simulink model "Disturbance"  (R2024b)
settings: Solver=FixedStepAuto  StartTime=0.0  StopTime=10.0  FixedStep=0.001  RelTol=1e-3
settings Model: Creator=abdal  LastModifiedBy=abdal

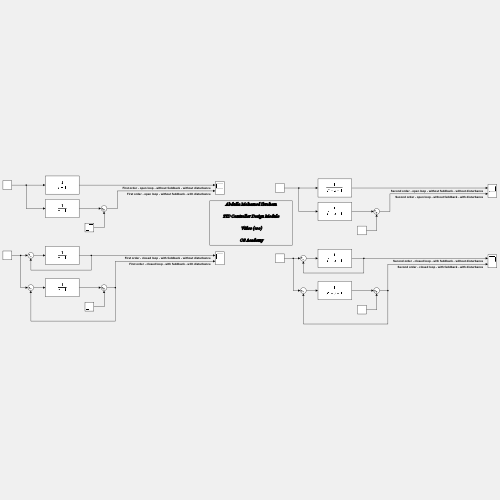
[thumbnail: Simulink's stored preview of the top-level diagram]
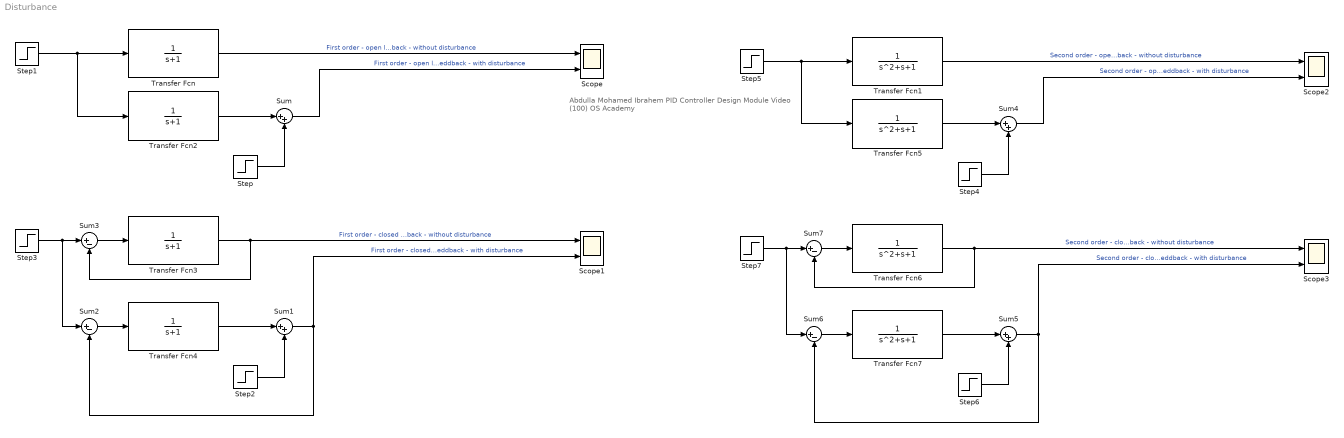
== system Disturbance ==
  note: Abdulla Mohamed Ibrahem
      | PID Controller Design Module
      | Video (100)
      | OS Academy
  Scope{,1..3} (4 alike) : Scope  NumInputPorts=2
  Step{,1..7} (8 alike) : Step  SampleTime=0
  Sum{,1,4..5} (4 alike) : Sum  Inputs=|++
  Sum{2..3,6..7} (4 alike) : Sum  Inputs=|+-
  Transfer Fcn{,2..4} (4 alike) : TransferFcn  Denominator=[1 1]
  Transfer Fcn{1,5..7} (4 alike) : TransferFcn  Denominator=[1 1 1]
  wires:
  Transfer Fcn/1 -> Scope/1  "First order - open loop - without feddback - without disturbance"
  Transfer Fcn2/1 -> Sum/1
  Sum/1 -> Scope/2  "First order - open loop - without feddback - with disturbance"
  Step/1 -> Sum/2
  Step1/1 -> Transfer Fcn/1, Transfer Fcn2/1
  Step3/1 -> Sum3/1, Sum2/1
  Step2/1 -> Sum1/2
  Sum1/1 -> Scope1/2, Sum2/2  "First order - closed loop - with feddback - with disturbance"
  Transfer Fcn4/1 -> Sum1/1
  Transfer Fcn3/1 -> Scope1/1, Sum3/2  "First order - closed loop - with feddback - without disturbance"
  Sum2/1 -> Transfer Fcn4/1
  Sum3/1 -> Transfer Fcn3/1
  Sum7/1 -> Transfer Fcn6/1
  Sum6/1 -> Transfer Fcn7/1
  Transfer Fcn6/1 -> Scope3/1, Sum7/2  "Second order - closed loop - with feddback - without disturbance"
  Transfer Fcn7/1 -> Sum5/1
  Sum5/1 -> Scope3/2, Sum6/2  "Second order - closed loop - with feddback - with disturbance"
  Step6/1 -> Sum5/2
  Step7/1 -> Sum6/1, Sum7/1
  Step5/1 -> Transfer Fcn5/1, Transfer Fcn1/1
  Step4/1 -> Sum4/2
  Sum4/1 -> Scope2/2  "Second order - open loop - without feddback - with disturbance"
  Transfer Fcn5/1 -> Sum4/1
  Transfer Fcn1/1 -> Scope2/1  "Second order - open loop - without feddback - without disturbance"
